simulink model "Lightning_McSeas_VCU_NEW_Speed_Mode"  (R2021b)
settings: Solver=FixedStepDiscrete  StartTime=0.0  StopTime=10.0  FixedStep=0.01  RelTol=1e-3  EnableMultiTasking=on
PreLoadFcn:
  | try, model_open; catch, disp('Error occurred while executing model pre-load callback: model_open.m'); disp('Please assure that the MATLAB working directory is set to the model directory before opening.'); end
InitFcn:
  | try, model_open; catch, end
undefined symbols (not defined in the file): dataName, enumName, enumValue, GCM, raptor_get_safe_string
libraries: Raptor_lib x71, simulink x8
(part 2 of 3)

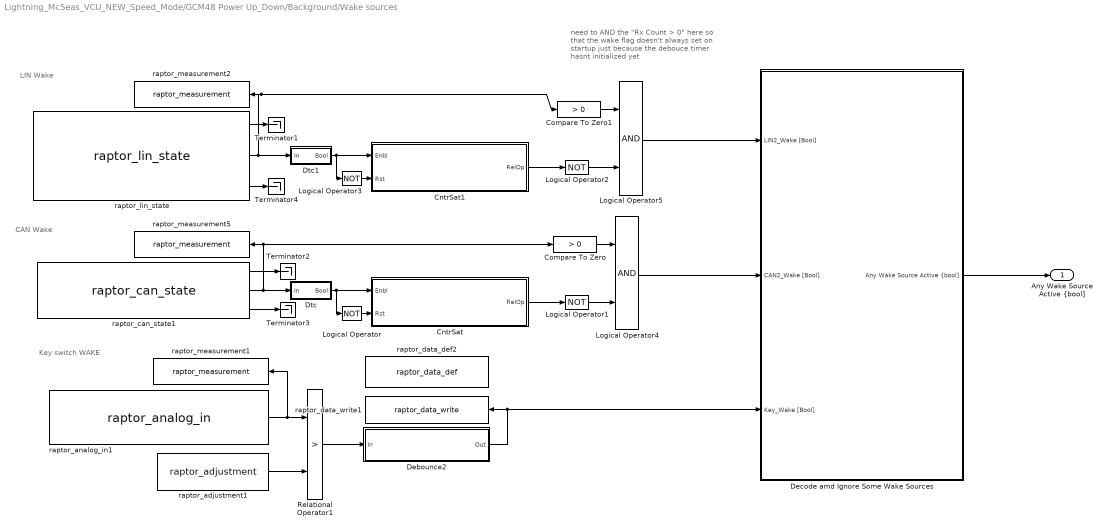
== system Lightning_McSeas_VCU_NEW_Speed_Mode/GCM48 Power Up_Down/Background/Wake sources ==
  note: CAN Wake
  note: Key switch WAKE
  note: LIN Wake
  note: need to AND the "Rx Count > 0" here so that the wake flag doesn't always set on startup just because the debouce timer hasnt initialized yet
  CntrSat : Subsystem  mask(CntrSat){init=0, inc=1, typ=uint32, relop=>=, th_nam='Wake_CAN2_SleepDelayTime', th_help='make sure this is long enough that we dont trigger a ton of EEPROM writes between messages', th_units='sec', th_gain=samptime, th_group=group}
      mask prompts: init "Initial Value (after a reset)"; inc "Increment"; typ "Data Type"; relop "Relational Operator"; th_nam "Thresh. Name"; th_help "Thresh. Help Text"; th_units "Thresh. Units"; th_gain "Thresh. Gain"; th_group "Thresh. Group"
      mask init: same as Lightning_McSeas_VCU_NEW_Speed_Mode/GCM48 Power Up_Down/Background/CntrSat2
      mask TypeOptions typ: double | single | int8 | uint8 | int16 | uint16 | int32 | uint32 | boolean
      mask TypeOptions relop: == | >= | >
      mask Display: disp(['Counter\n' typ '\n' relop ' ' th_nam]);
  CntrSat1 : Subsystem  mask(CntrSat){init=0, inc=1, typ=uint32, relop=>=, th_nam='Wake_LIN2_SleepDelayTime', th_help='make sure this is long enough that we dont trigger a ton of EEPROM writes between messages', th_units='sec', th_gain=samptime, th_group=group}
      mask prompts: init "Initial Value (after a reset)"; inc "Increment"; typ "Data Type"; relop "Relational Operator"; th_nam "Thresh. Name"; th_help "Thresh. Help Text"; th_units "Thresh. Units"; th_gain "Thresh. Gain"; th_group "Thresh. Group"
      mask init: same as Lightning_McSeas_VCU_NEW_Speed_Mode/GCM48 Power Up_Down/Background/CntrSat2
      mask TypeOptions typ: double | single | int8 | uint8 | int16 | uint16 | int32 | uint32 | boolean
      mask TypeOptions relop: == | >= | >
      mask Display: disp(['Counter\n' typ '\n' relop ' ' th_nam]);
  Compare To Zero : simulink/Logic and Bit Operations/Compare To Zero  relop=>  OutDataTypeStr=boolean
  Compare To Zero1 : simulink/Logic and Bit Operations/Compare To Zero  relop=>  OutDataTypeStr=boolean
  Debounce2 : Subsystem
  Decode amd Ignore Some Wake Sources : Subsystem
  Dtc : Subsystem  mask(Dtc){init=0, relop===}
      mask prompts: init "Initial Condition (of input):"; relop "Relational Operator"
      mask init:
      | cb = gcb;
      | 
      | % --- Parameter Setting
      | set_param([cb '/Relational Operator'], 'Operator', relop);
      mask TypeOptions relop: == | ~= | < | <= | >= | >
      mask Display: disp(['U ' relop ' U/z']);
  Dtc1 : Subsystem  mask(Dtc){init=0, relop===}
      mask prompts: init "Initial Condition (of input):"; relop "Relational Operator"
      mask init:
      | cb = gcb;
      | 
      | % --- Parameter Setting
      | set_param([cb '/Relational Operator'], 'Operator', relop);
      mask TypeOptions relop: == | ~= | < | <= | >= | >
      mask Display: disp(['U ' relop ' U/z']);
  Logical Operator{,1..3} (4 alike) : Logic  Operator=NOT  AllPortsSameDT=off  OutDataTypeStr=boolean
  Logical Operator4 : Logic  AllPortsSameDT=off  OutDataTypeStr=boolean
  Logical Operator5 : Logic  AllPortsSameDT=off  OutDataTypeStr=boolean
  Relational Operator1 : RelationalOperator  Operator=>  OutDataTypeStr=boolean  RndMeth=Simplest
  Terminator{1..4} (4 alike) : Terminator
  raptor_adjustment1 : Raptor_lib/Data Storage/raptor_adjustment  paramName='WAKE_INPUT1_Threshold'  nameSource=Parameter  initValue=1200  dataType=uint16  storage=NonVolatile (EEPROM)  calDispType=Number  calEnum={'False', 'True'}  calGain=1  calOffset=0.0  calMax=inf  calMin=-inf  calFormat='-1'  calUnit='V'  calHelp='The value of WAKE_INPUT1 analog to set key switch to true.'  calAccess=4  calFunction=group  calDispHeaders=off  calColHeaders={'Col1' 'Col2' 'Col3'}  calRowHeaders={'Row1' 'Row2' 'Row3'}
      settings: SourceProductName=Raptor
  raptor_analog_in1 : Raptor_lib/Input & Output/raptor_analog_in  resourceValues=DG1|DG2|DG3|DG4|AN1|AN2|AN3|AN4|AN5|AN6|AN7|AN8|AN9|AN10|AN11|AN12|WAKE_INPUT1|(None)  resource=WAKE_INPUT1  pullUDValues=[]  pullUD=[]  rangeValues=[]  range=[]  filterrateValues=[]  filterrate='RAPTOR MASK DEFAULT'  resolutionValues=[]  resolution=[]
      settings: SourceProductName=Raptor
  raptor_can_state1 : Raptor_lib/CAN/raptor_can_state  resourceValues=CAN1|CAN2|CAN3|CAN4|CAN5|CAN6|(None)  resource=CAN2  errOut='RAPTOR MASK DEFAULT'
      settings: SourceProductName=Raptor
  raptor_data_def2 : Raptor_lib/Data Storage/raptor_data_def  dataName='KeySw_Bgnd'  initValue=0  dataType=boolean  storage=Volatile (RAM)  calVisible=on  calType=Measurement  calDispType=Number  calEnum={'False', 'True'}  calGain=1.0  calOffset=0  calMin=-Inf  calMax=Inf  calFormat='-1'  calUnit='Bool'  calHelp='Key switch reading from background task'  calAccess=4  calFunction=group  calDispHeaders=off  calColHeaders={'Col1' 'Col2' 'Col3'}  calRowHeaders={'Row1' 'Row2' 'Row3'}
      settings: SourceProductName=Raptor
  raptor_data_write1 : Raptor_lib/Data Storage/raptor_data_write  dataName='KeySw_Bgnd'  dataShape=Scalar  idxSource=Input Port  idxRow=1  idxCol=1
      settings: SourceProductName=Raptor
  raptor_lin_state : Raptor_lib/LIN/raptor_lin_state  linBus='LIN2'
      settings: SourceProductName=Raptor
  raptor_measurement1 : Raptor_lib/Data Storage/raptor_measurement  paramName='Wake_INPUT1_Vlts'  nameSource=Parameter  calDispType=Number  calEnum={'False', 'True'}  calGain=38/4096  calOffset=0.0  calMax=inf  calMin=-inf  calFormat='-1'  calUnit=''  calHelp=''  calAccess=4  calFunction=group  calVisible=on
      settings: SourceProductName=Raptor
  raptor_measurement2 : Raptor_lib/Data Storage/raptor_measurement  paramName='Wake_LIN2_RxCount'  nameSource=Parameter  calDispType=Number  calEnum={'False', 'True'}  calGain=1.0  calOffset=0.0  calMax=inf  calMin=-inf  calFormat='-1'  calUnit=''  calHelp=''  calAccess=4  calFunction=group  calVisible=on
      settings: SourceProductName=Raptor
  raptor_measurement5 : Raptor_lib/Data Storage/raptor_measurement  paramName='Wake_CAN2_RxCount'  nameSource=Parameter  calDispType=Number  calEnum={'False', 'True'}  calGain=1.0  calOffset=0.0  calMax=inf  calMin=-inf  calFormat='-1'  calUnit=''  calHelp=''  calAccess=4  calFunction=group  calVisible=on
      settings: SourceProductName=Raptor
  "Any Wake Source Active {bool]" : Outport  VectorParamsAs1DForOutWhenUnconnected=off
  wires:
  Logical Operator5/1 -> Decode amd Ignore Some Wake Sources/1(LIN2_Wake [Bool])
  Logical Operator2/1 -> Logical Operator5/2
  Compare To Zero1/1 -> Logical Operator5/1
  Logical Operator4/1 -> Decode amd Ignore Some Wake Sources/2(CAN2_Wake [Bool])
  Compare To Zero/1 -> Logical Operator4/1
  Logical Operator1/1 -> Logical Operator4/2
  Decode amd Ignore Some Wake Sources/1("Any Wake Source Active {bool]") -> "Any Wake Source Active {bool]"/1
  raptor_can_state1/3 -> Terminator3/1
  raptor_adjustment1/1 -> Relational Operator1/2
  raptor_can_state1/1 -> Terminator2/1
  raptor_lin_state/3 -> Terminator4/1
  raptor_lin_state/1 -> Terminator1/1
  CntrSat1/1(RelOp) -> Logical Operator2/1
  Logical Operator/1 -> CntrSat/2(Rst)
  raptor_lin_state/2 -> Dtc1/1(In), raptor_measurement2/1, Compare To Zero1/1
  Logical Operator3/1 -> CntrSat1/2(Rst)
  Dtc1/1(Bool) -> Logical Operator3/1, CntrSat1/1(Enbl)
  Relational Operator1/1 -> Debounce2/1(In)
  Dtc/1(Bool) -> CntrSat/1(Enbl), Logical Operator/1
  CntrSat/1(RelOp) -> Logical Operator1/1
  raptor_analog_in1/1 -> Relational Operator1/1, raptor_measurement1/1
  Debounce2/1(Out) -> raptor_data_write1/1, Decode amd Ignore Some Wake Sources/3(Key_Wake [Bool])
  raptor_can_state1/2 -> raptor_measurement5/1, Compare To Zero/1, Dtc/1(In)

== system Lightning_McSeas_VCU_NEW_Speed_Mode/Foreground/CAN/RC Rx/Actuators ==
  note: This subsystem isnt correct****
  note: -might be able to just combine back actuators to same thing - or they might be inversers of each other
  Rise of Back : Inport
  Rise of Front : Inport  Port=2
  Gain1 : Gain  Gain=51
  Gain2 : Gain  Gain=51
  If statement for on off switch1 : Subsystem  Commented=on
  Subsystem : Subsystem  Commented=on
  raptor_can_txmsg3 : Raptor_lib/CAN/raptor_can_txmsg  canDefinition=struct('dbcFile', 'actuator_atmpt1.dbc','message', 'actuator3','comment', '','signals', {{'position_send3'}},'enabled', [ 1;],'scaled', [ 1;],'canBus', '''CAN1''','messageID', [ 32;],'idMask', [ 536870911;],'payloadMask', [],'payloadValue', [],'period', [ 0;],'mailbox', '','queueSize', [ 1;],'label', [ 0;],'ver', [ 2;],'showID', [ 0;],'showRaw', [ 0;],'showRawMsg', [ 0;],'fill', [ 0;],'editID', [ 0;],'signalOrder', [ 1;],'signalAscDes', [ 1;])  canBus='CAN1'  queueSize=1  payloadMask=[]  payloadValue=[]  period=0  showID=0  label=0  idMask=hex2dec('1FFFFFFF')  fill=0  id=32  showRaw=0  signalOrder=1  signalInfo={{struct('Name', 'position_send3','Startbit', [ 0;],'SignalSize', [ 16;],'ByteOrder', 'LittleEndian','ValueType', 'UNSIGNED','Class', 'uint16','Signed', [ 0;],'Factor', [ 1;],'Offset', [ 0;],'Min', [ 0;],'Max', [ 0;],'Units', '','Comment', '','StartBit', [ 0;])}}
      settings: SourceProductName=Raptor
  raptor_can_txmsg4 : Raptor_lib/CAN/raptor_can_txmsg  canDefinition=struct('dbcFile', 'actuator_atmpt1.dbc','message', 'actuator2','comment', '','signals', {{'position_send2'}},'enabled', [ 1;],'scaled', [ 1;],'canBus', '''CAN1''','messageID', [ 31;],'idMask', [ 536870911;],'payloadMask', [],'payloadValue', [],'period', [ 0;],'mailbox', '','queueSize', [ 1;],'label', [ 0;],'ver', [ 2;],'showID', [ 0;],'showRaw', [ 0;],'showRawMsg', [ 0;],'fill', [ 0;],'editID', [ 0;],'signalOrder', [ 1;],'signalAscDes', [ 1;])  canBus='CAN1'  queueSize=1  payloadMask=[]  payloadValue=[]  period=0  showID=0  label=0  idMask=hex2dec('1FFFFFFF')  fill=0  id=31  showRaw=0  signalOrder=1  signalInfo={{struct('Name', 'position_send2','Startbit', [ 0;],'SignalSize', [ 16;],'ByteOrder', 'LittleEndian','ValueType', 'UNSIGNED','Class', 'uint16','Signed', [ 0;],'Factor', [ 1;],'Offset', [ 0;],'Min', [ 0;],'Max', [ 0;],'Units', '','Comment', '','StartBit', [ 0;])}}
      settings: SourceProductName=Raptor
  wires:
  Rise of Back/1 -> Gain2/1
  Gain2/1 -> raptor_can_txmsg4/1
  Gain1/1 -> raptor_can_txmsg3/1
  Rise of Front/1 -> Gain1/1

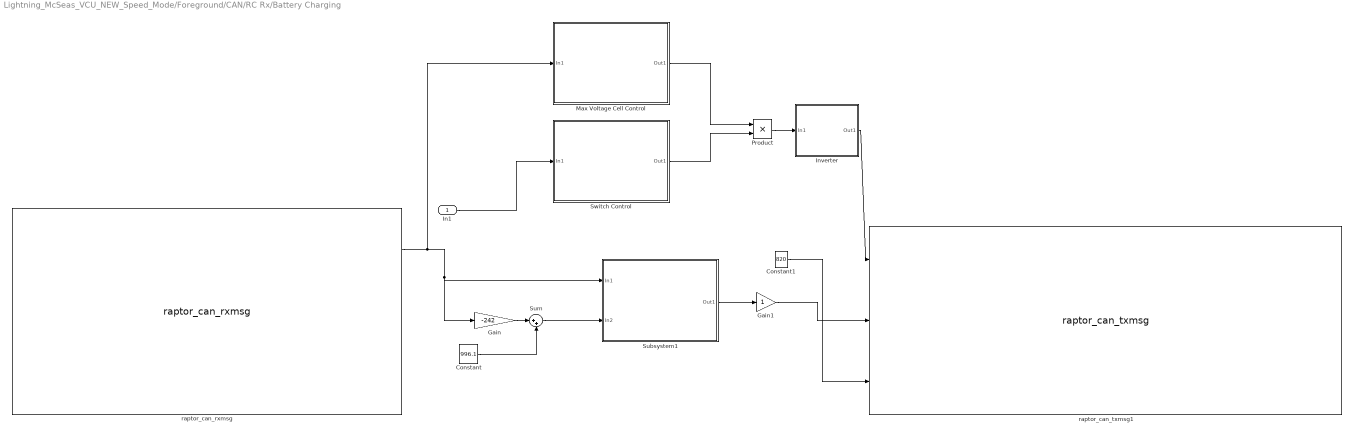
== system Lightning_McSeas_VCU_NEW_Speed_Mode/Foreground/CAN/RC Rx/Battery Charging ==
  In1 : Inport
  Constant : Constant  Value=996.1
  Constant1 : Constant  Value=820
  Gain : Gain  Gain=-242
  Gain1 : Gain
  Inverter : Subsystem
  Max Voltage Cell Control : Subsystem
  Product : Product
  Subsystem1 : Subsystem
  Sum : Sum  Inputs=|++
  Switch Control : Subsystem
  raptor_can_rxmsg : Raptor_lib/CAN/raptor_can_rxmsg  canDefinition=struct('dbcFile', 'BCM_VehBus_StdInterface.dbc','message', 'BCM_Meas_A','comment', '','signals', {{'bcm_cell_vmax_a','bcm_cell_vmin_a','bcm_i_lem_a','bcm_vbat_a','bcm_vbus_a','bcm_vfuse_a'}},'enabled', [ 1 1 1 1 1 1;],'scaled', [ 1 1 1 1 1 1;],'canBus', '''CAN1''','messageID', [ 1072;],'idMask', [ 536870911;],'payloadMask', [],'payloadValue', [],'period', [ 0;],'mailbox', '''''','queueSize', [ 1;],'label', [ 0;],'ver', [ 2;],'showID', [ 0;],'showRaw', [ 0;],'showRawMsg', [ 0;],'showAge', [ 1;],'fill', [ 0;],'editID', [ 0;],'signalOrder', [ 1;],'signalAscDes', [ 1;])  canBus='CAN1'  mailbox=''  payloadMask=[]  payloadValue=[]  idMask=hex2dec('1FFFFFFF')  queueSize=1  showID=0  label=0  fill=0  id=1072  showRaw=0  showAge=1  signalOrder=1  signalInfo={{struct('Name', 'bcm_cell_vmin_a','Startbit', [ 0;],'SignalSize', [ 12;],'ByteOrder', 'BigEndian','ValueType', 'UNSIGNED','Class', 'uint16','Signed', [ 0;],'Factor', [ 0.002;],'Offset', [ 0;],'Min', [ 0;],'Max', [ 5;],'Units', 'volts','Comment', 'Min cell voltage.','StartBit', [ 56;]),struct('Name', 'bcm_cell_vmax_a','Startbit', [ 0;],'SignalSize', [ 12;],'ByteOrder', 'BigEndian','ValueType', 'UNSIGNED','Class', 'uint16','Signed', [ 0;],'Factor', [ 0.002;],'Offset', [ 0;],'Min', [ 0;],'Max', [ 5;],'Units', 'volts','Comment', 'Max cell voltage.','StartBit', [ 52;]),struct('Name', 'bcm_vfuse_a','Startbit', [ 0;],'SignalSize', [ 8;],'ByteOrder', 'BigEndian','ValueType', 'UNSIGNED','Class', 'uint8','Signed', [ 0;],'Factor', [ 0.5;],'Offset', [ 0;],'Min', [ 0;],'Max', [ 125;],'Units', 'volts','Comment', 'HV bus positive voltage measurement.','StartBit', [ 24;]),struct('Name', 'bcm_vbus_a','Startbit', [ 0;],'SignalSize', [ 8;],'ByteOrder', 'BigEndian','ValueType', 'UNSIGNED','Class', 'uint8','Signed', [ 0;],'Factor', [ 0.5;],'Offset', [ 0;],'Min', [ 0;],'Max', [ 125;],'Units', 'volts','Comment', 'HV bus positive voltage measurement.','StartBit', [ 32;]),struct('Name', 'bcm_vbat_a','Startbit', [ 0;],'SignalSize', [ 8;],'ByteOrder', 'BigEndian','ValueType', 'UNSIGNED','Class', 'uint8','Signed', [ 0;],'Factor', [ 0.5;],'Offset', [ 0;],'Min', [ 0;],'Max', [ 125;],'Units', 'volts','Comment', 'HV bus positive voltage measurement.','StartBit', [ 16;]),struct('Name', 'bcm_i_lem_a','Startbit', [ 0;],'SignalSize', [ 16;],'ByteOrder', 'BigEndian','ValueType', 'UNSIGNED','Class', 'uint16','Signed', [ 0;],'Factor', [ 0.025;],'Offset', [ -1000;],'Min', [ -1000;],'Max', [ 500;],'Units', 'amps','Comment', '[Development Sensor] HV Battery Current where negative is battery discharge and positive is battery charge.','StartBit', [ 8;])}}  showRawMsg=0
      settings: SourceProductName=Raptor
  raptor_can_txmsg1 : Raptor_lib/CAN/raptor_can_txmsg  canDefinition=struct('dbcFile', 'Elcon_Charger.dbc','message', 'Charger_Request','comment', '','signals', {{'charger_control','charger_max_current','charger_max_voltage'}},'enabled', [ 1 1 1;],'scaled', [ 1 1 1;],'canBus', '''CAN1''','messageID', [ 403105268;],'idMask', [ 536870911;],'payloadMask', [],'payloadValue', [],'period', [ 0;],'mailbox', '','queueSize', [ 1;],'label', [ 0;],'ver', [ 2;],'showID', [ 0;],'showRaw', [ 0;],'showRawMsg', [ 0;],'fill', [ 0;],'editID', [ 0;],'signalOrder', [ 1;],'signalAscDes', [ 1;])  canBus='CAN1'  queueSize=1  payloadMask=[]  payloadValue=[]  period=0  showID=0  label=0  idMask=hex2dec('1FFFFFFF')  fill=0  id=403105268  showRaw=0  signalOrder=1  signalInfo={{struct('Name', 'charger_max_voltage','Startbit', [ 0;],'SignalSize', [ 16;],'ByteOrder', 'BigEndian','ValueType', 'UNSIGNED','Class', 'uint16','Signed', [ 0;],'Factor', [ 0.1;],'Offset', [ 0;],'Min', [ 0;],'Max', [ 0;],'Units', 'V','Comment', 'Max Allowable Charging Terminal Voltage','StartBit', [ 8;]),struct('Name', 'charger_max_current','Startbit', [ 0;],'SignalSize', [ 16;],'ByteOrder', 'BigEndian','ValueType', 'UNSIGNED','Class', 'uint16','Signed', [ 0;],'Factor', [ 0.1;],'Offset', [ 0;],'Min', [ 0;],'Max', [ 0;],'Units', 'A','Comment', 'Max Allowable Charging Current','StartBit', [ 24;]),struct('Name', 'charger_control','Startbit', [ 0;],'SignalSize', [ 8;],'ByteOrder', 'LittleEndian','ValueType', 'UNSIGNED','Class', 'uint8','Signed', [ 0;],'Factor', [ 1;],'Offset', [ 0;],'Min', [ 0;],'Max', [ 0;],'Units', '','Comment', 'Toggle charging','StartBit', [ 32;])}}
      settings: SourceProductName=Raptor
  wires:
  In1/1 -> Switch Control/1(In1)
  Gain/1 -> Sum/1
  Subsystem1/1(Out1) -> Gain1/1
  Constant1/1 -> raptor_can_txmsg1/3
  Constant/1 -> Sum/2
  Sum/1 -> Subsystem1/2(In2)
  Switch Control/1(Out1) -> Product/2
  Max Voltage Cell Control/1(Out1) -> Product/1
  Gain1/1 -> raptor_can_txmsg1/2
  raptor_can_rxmsg/2 -> Max Voltage Cell Control/1(In1), Gain/1, Subsystem1/1(In1)
  Product/1 -> Inverter/1(In1)
  Inverter/1(Out1) -> raptor_can_txmsg1/1

== system Lightning_McSeas_VCU_NEW_Speed_Mode/Foreground/CAN/RC Rx/Battery Switch ==
  value in : Inport
  Constant : Constant  Commented=on  Value=10000  OutDataTypeStr=uint16
  Constant1 : Constant  Commented=on  Value=100  OutDataTypeStr=uint32
  If statement for on off switch : Subsystem
  If statement for on off switch1 : Subsystem  Commented=on
  If statement for on off switch2 : Subsystem
  raptor_can_txmsg : Raptor_lib/CAN/raptor_can_txmsg  canDefinition=struct('dbcFile', 'BCM_VehBus_StdInterface.dbc','message', 'BCM_Request','comment', '','signals', {{'hsc_bcm_enable','hsc_bcm_epo','hsc_bcm_leakage_ena','hsc_bcm_mainc_close'}},'enabled', [ 1 1 1 1;],'scaled', [ 1 1 1 1;],'canBus', '''CAN1''','messageID', [ 1024;],'idMask', [ 536870911;],'payloadMask', [],'payloadValue', [],'period', [ 0;],'mailbox', '','queueSize', [ 1;],'label', [ 0;],'ver', [ 2;],'showID', [ 0;],'showRaw', [ 0;],'showRawMsg', [ 0;],'fill', [ 0;],'editID', [ 0;],'signalOrder', [ 1;],'signalAscDes', [ 1;])  canBus='CAN1'  queueSize=1  payloadMask=[]  payloadValue=[]  period=0  showID=0  label=0  idMask=hex2dec('1FFFFFFF')  fill=0  id=1024  showRaw=0  signalOrder=1  signalInfo={{struct('Name', 'hsc_bcm_mainc_close','Startbit', [ 0;],'SignalSize', [ 1;],'ByteOrder', 'BigEndian','ValueType', 'UNSIGNED','Class', 'uint8','Signed', [ 0;],'Factor', [ 1;],'Offset', [ 0;],'Min', [ 0;],'Max', [ 1;],'Units', 'flag','Comment', 'Vehicle main contactor command.','StartBit', [ 2;]),struct('Name', 'hsc_bcm_leakage_ena','Startbit', [ 0;],'SignalSize', [ 1;],'ByteOrder', 'BigEndian','ValueType', 'UNSIGNED','Class', 'uint8','Signed', [ 0;],'Factor', [ 1;],'Offset', [ 0;],'Min', [ 0;],'Max', [ 1;],'Units', 'flag','Comment', 'Vehicle leakage detection enabled (bcm_gfd calculation).','StartBit', [ 3;]),struct('Name', 'hsc_bcm_epo','Startbit', [ 0;],'SignalSize', [ 1;],'ByteOrder', 'BigEndian','ValueType', 'UNSIGNED','Class', 'uint8','Signed', [ 0;],'Factor', [ 1;],'Offset', [ 0;],'Min', [ 0;],'Max', [ 1;],'Units', 'flag','Comment', 'Vehicle Emergency Power Off command, fast shutdown.','StartBit', [ 1;]),struct('Name', 'hsc_bcm_enable','Startbit', [ 0;],'SignalSize', [ 1;],'ByteOrder', 'BigEndian','ValueType', 'UNSIGNED','Class', 'uint8','Signed', [ 0;],'Factor', [ 1;],'Offset', [ 0;],'Min', [ 0;],'Max', [ 1;],'Units', 'flag','Comment', 'Flag from vehicle controller allowing BCM to accept commands.','StartBit', [ 0;])}}
      settings: SourceProductName=Raptor
  raptor_pwm_out : Raptor_lib/Input & Output/raptor_pwm_out  Commented=on  showEnable=1  resourceValues=LSO1|LSO2|LSO3|LSO4|LSO5|LSO6|LSO7|LSO8|(None)  resource=LSO2  driverTypeValues=Low Side  driverType=Low Side
      settings: SourceProductName=Raptor
  wires:
  value in/1 -> If statement for on off switch2/1(value in), If statement for on off switch/1(value in)
  If statement for on off switch2/1(Value out) -> raptor_can_txmsg/1
  If statement for on off switch1/1(Value out) -> raptor_pwm_out/1
  Constant1/1 -> raptor_pwm_out/3
  Constant/1 -> raptor_pwm_out/2
  If statement for on off switch/1(Value out) -> raptor_can_txmsg/4

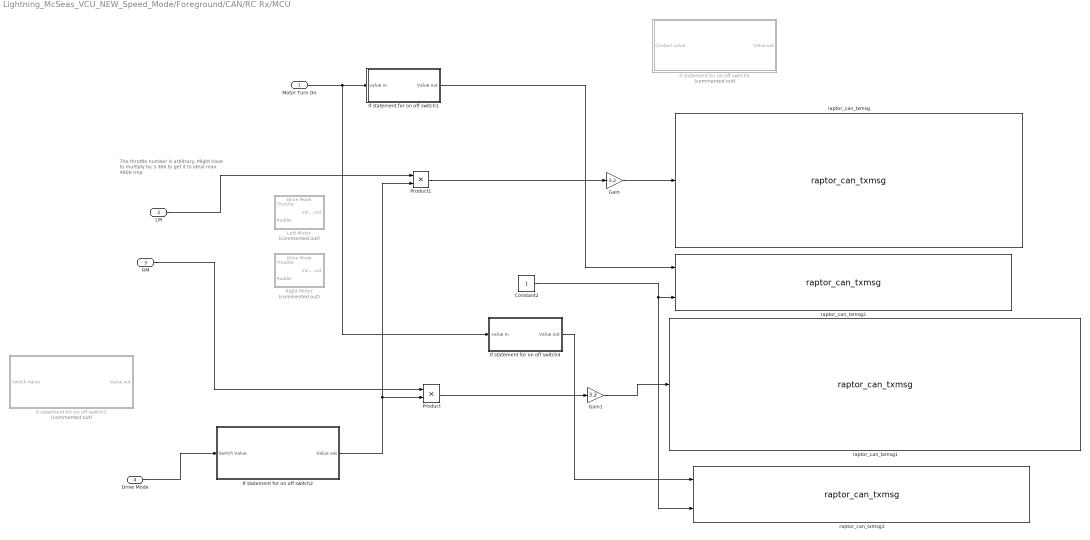
== system Lightning_McSeas_VCU_NEW_Speed_Mode/Foreground/CAN/RC Rx/MCU ==
  note: The throttle number is arbitrary. Might have to multiply by 3.366 to get it to ideal max 4800 rmp
  Motor Turn On : Inport
  LM : Inport  Port=2
  RM : Inport  Port=3
  Drive Mode : Inport  Port=4
  Constant2 : Constant
  Gain : Gain  Gain=-3.2
  Gain1 : Gain  Gain=3.2
  If statement for on off switch1 : Subsystem
  If statement for on off switch2 : Subsystem
  If statement for on off switch3 : Subsystem  Commented=on
  If statement for on off switch4 : Subsystem
  If statement for on off switch5 : Subsystem  Commented=on
  Left Motor : Subsystem  Commented=on
      settings: PortSchema="{\"entries\":[{\"content\":{\"sides\":[{\"content\":{\"connectorIds\":[\"In1\",\"In2\"]},\"type\":\"ConnectorPlacement.EquallySpacedRectSide\",\"uuid\":\"2083280e-5025-4497-a6f4-d95150e30dec\"},{\"content\":{\"connectorIds\":[\"Out1\"],\"side\":\"RIGHT\"},\"type\":\"ConnectorPlacement.EquallySpacedRectSide\",\"uuid\":\"61c851a0-d108-4419-a7df-f59beb96b75c\"},{\"content\":{\"connectorIds\":[\"In3\"],\"side\":\"TOP\"},\"type\":\"ConnectorPlacement.EquallySpacedRectSide\",\"uuid\":\"d9cef341-ca3e-4785-954e-89a8b6a8f97d\"}]},\"type\":\"ConnectorPlacement.EquallySpacedConnector\",\"uuid\":\"5877ad35-291b-4063-ae6a-1f18cb91c1ea\"}],\"packageUris\":[\"http://schema.mathworks.com/mf0/Connector/R2020b\"],\"version\":\"1.0\"}"
  Product : Product
  Product1 : Product
  Right Motor : Subsystem  Commented=on
      settings: PortSchema="{\"entries\":[{\"content\":{\"sides\":[{\"content\":{\"connectorIds\":[\"In1\",\"In2\"]},\"type\":\"ConnectorPlacement.EquallySpacedRectSide\",\"uuid\":\"2083280e-5025-4497-a6f4-d95150e30dec\"},{\"content\":{\"connectorIds\":[\"Out1\"],\"side\":\"RIGHT\"},\"type\":\"ConnectorPlacement.EquallySpacedRectSide\",\"uuid\":\"61c851a0-d108-4419-a7df-f59beb96b75c\"},{\"content\":{\"connectorIds\":[\"In3\"],\"side\":\"TOP\"},\"type\":\"ConnectorPlacement.EquallySpacedRectSide\",\"uuid\":\"d9cef341-ca3e-4785-954e-89a8b6a8f97d\"}]},\"type\":\"ConnectorPlacement.EquallySpacedConnector\",\"uuid\":\"5877ad35-291b-4063-ae6a-1f18cb91c1ea\"}],\"packageUris\":[\"http://schema.mathworks.com/mf0/Connector/R2020b\"],\"version\":\"1.0\"}"
  raptor_can_txmsg : Raptor_lib/CAN/raptor_can_txmsg  canDefinition=struct('dbcFile', 'A1_MICH_EV_BOAT.dbc','message', 'command1','comment', '','signals', {{'throttleCurrent1'}},'enabled', [ 1;],'scaled', [ 1;],'canBus', '''CAN1''','messageID', [ 550;],'idMask', [ 536870911;],'payloadMask', [],'payloadValue', [],'period', [ 0;],'mailbox', '','queueSize', [ 1;],'label', [ 0;],'ver', [ 2;],'showID', [ 0;],'showRaw', [ 0;],'showRawMsg', [ 0;],'fill', [ 0;],'editID', [ 0;],'signalOrder', [ 1;],'signalAscDes', [ 1;])  canBus='CAN1'  queueSize=1  payloadMask=[]  payloadValue=[]  period=0  showID=0  label=0  idMask=hex2dec('1FFFFFFF')  fill=0  id=550  showRaw=0  signalOrder=1  signalInfo={{struct('Name', 'throttleCurrent1','Startbit', [ 0;],'SignalSize', [ 16;],'ByteOrder', 'LittleEndian','ValueType', 'SIGNED','Class', 'int16','Signed', [ 1;],'Factor', [ 1;],'Offset', [ 0;],'Min', [ 0;],'Max', [ 0;],'Units', '','Comment', '','StartBit', [ 0;])}}
      settings: SourceProductName=Raptor
  raptor_can_txmsg1 : Raptor_lib/CAN/raptor_can_txmsg  canDefinition=struct('dbcFile', 'A1_MICH_EV_BOAT.dbc','message', 'command1','comment', '','signals', {{'throttleCurrent1'}},'enabled', [ 1;],'scaled', [ 1;],'canBus', '''CAN1''','messageID', [ 550;],'idMask', [ 536870911;],'payloadMask', [],'payloadValue', [],'period', [ 0;],'mailbox', '','queueSize', [ 1;],'label', [ 0;],'ver', [ 2;],'showID', [ 0;],'showRaw', [ 0;],'showRawMsg', [ 0;],'fill', [ 0;],'editID', [ 0;],'signalOrder', [ 1;],'signalAscDes', [ 1;])  canBus='CAN1'  queueSize=1  payloadMask=[]  payloadValue=[]  period=0  showID=0  label=0  idMask=hex2dec('1FFFFFFF')  fill=0  id=550  showRaw=0  signalOrder=1  signalInfo={{struct('Name', 'throttleCurrent1','Startbit', [ 0;],'SignalSize', [ 16;],'ByteOrder', 'LittleEndian','ValueType', 'SIGNED','Class', 'int16','Signed', [ 1;],'Factor', [ 1;],'Offset', [ 0;],'Min', [ 0;],'Max', [ 0;],'Units', '','Comment', '','StartBit', [ 0;])}}
      settings: SourceProductName=Raptor
  raptor_can_txmsg2 : Raptor_lib/CAN/raptor_can_txmsg  canDefinition=struct('dbcFile', 'A1_MICH_EV_BOAT.dbc','message', 'NMT','comment', '','signals', {{'id','o1'}},'enabled', [ 1 1;],'scaled', [ 1 1;],'canBus', '''CAN1''','messageID', [ 0;],'idMask', [ 536870911;],'payloadMask', [],'payloadValue', [],'period', [ 0;],'mailbox', '','queueSize', [ 1;],'label', [ 0;],'ver', [ 2;],'showID', [ 0;],'showRaw', [ 0;],'showRawMsg', [ 0;],'fill', [ 0;],'editID', [ 0;],'signalOrder', [ 1;],'signalAscDes', [ 1;])  canBus='CAN1'  queueSize=1  payloadMask=[]  payloadValue=[]  period=0  showID=0  label=0  idMask=hex2dec('1FFFFFFF')  fill=0  id=0  showRaw=0  signalOrder=1  signalInfo={{struct('Name', 'id','Startbit', [ 0;],'SignalSize', [ 8;],'ByteOrder', 'LittleEndian','ValueType', 'UNSIGNED','Class', 'uint8','Signed', [ 0;],'Factor', [ 1;],'Offset', [ 0;],'Min', [ 0;],'Max', [ 0;],'Units', '','Comment', 'controller id hex (0x26 or 0x27 in our case)','StartBit', [ 8;]),struct('Name', 'o1','Startbit', [ 0;],'SignalSize', [ 8;],'ByteOrder', 'LittleEndian','ValueType', 'UNSIGNED','Class', 'uint8','Signed', [ 0;],'Factor', [ 1;],'Offset', [ 0;],'Min', [ 0;],'Max', [ 0;],'Units', '','Comment', 'value 01 hex','StartBit', [ 0;])}}
      settings: SourceProductName=Raptor
  raptor_can_txmsg3 : Raptor_lib/CAN/raptor_can_txmsg  canDefinition=struct('dbcFile', 'A1_MICH_EV_BOAT.dbc','message', 'NMT','comment', '','signals', {{'id','o1'}},'enabled', [ 1 1;],'scaled', [ 1 1;],'canBus', '''CAN1''','messageID', [ 0;],'idMask', [ 536870911;],'payloadMask', [],'payloadValue', [],'period', [ 0;],'mailbox', '','queueSize', [ 1;],'label', [ 0;],'ver', [ 2;],'showID', [ 0;],'showRaw', [ 0;],'showRawMsg', [ 0;],'fill', [ 0;],'editID', [ 0;],'signalOrder', [ 1;],'signalAscDes', [ 1;])  canBus='CAN1'  queueSize=1  payloadMask=[]  payloadValue=[]  period=0  showID=0  label=0  idMask=hex2dec('1FFFFFFF')  fill=0  id=0  showRaw=0  signalOrder=1  signalInfo={{struct('Name', 'id','Startbit', [ 0;],'SignalSize', [ 8;],'ByteOrder', 'LittleEndian','ValueType', 'UNSIGNED','Class', 'uint8','Signed', [ 0;],'Factor', [ 1;],'Offset', [ 0;],'Min', [ 0;],'Max', [ 0;],'Units', '','Comment', 'controller id hex (0x26 or 0x27 in our case)','StartBit', [ 8;]),struct('Name', 'o1','Startbit', [ 0;],'SignalSize', [ 8;],'ByteOrder', 'LittleEndian','ValueType', 'UNSIGNED','Class', 'uint8','Signed', [ 0;],'Factor', [ 1;],'Offset', [ 0;],'Min', [ 0;],'Max', [ 0;],'Units', '','Comment', 'value 01 hex','StartBit', [ 0;])}}
      settings: SourceProductName=Raptor
  wires:
  Motor Turn On/1 -> If statement for on off switch4/1(value in), If statement for on off switch1/1(value in)
  RM/1 -> Product/1
  LM/1 -> Product1/1
  Product/1 -> Gain1/1
  Product1/1 -> Gain/1
  If statement for on off switch2/1(Value out) -> Product1/2, Product/2
  Drive Mode/1 -> If statement for on off switch2/1(Switch Value)
  Gain/1 -> raptor_can_txmsg/1
  Gain1/1 -> raptor_can_txmsg1/1
  If statement for on off switch1/1(Value out) -> raptor_can_txmsg2/1
  Constant2/1 -> raptor_can_txmsg3/2, raptor_can_txmsg2/2
  If statement for on off switch4/1(Value out) -> raptor_can_txmsg3/1

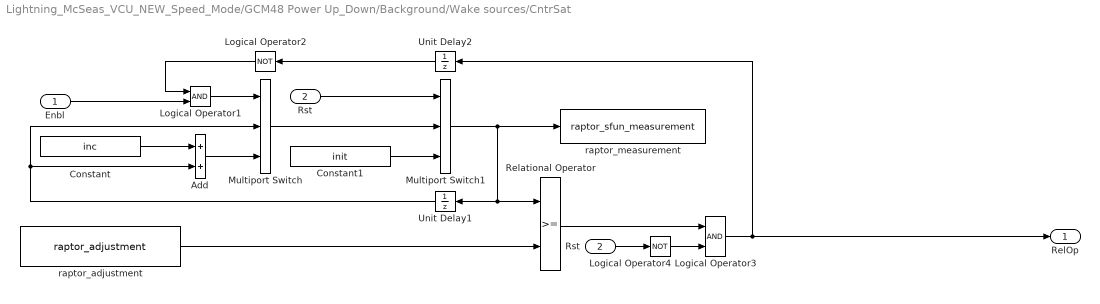
== system Lightning_McSeas_VCU_NEW_Speed_Mode/GCM48 Power Up_Down/Background/Wake sources/CntrSat ==
  Enbl : Inport
  Rst : Inport  Port=2
  Add : Sum  InputSameDT=on  OutDataTypeStr=Inherit: Same as first input
  Constant : Constant  Value=inc  OutDataTypeStr=uint32
  Constant1 : Constant  Value=init  OutDataTypeStr=uint32
  Logical Operator1 : Logic  OutDataTypeStr=boolean
  Logical Operator2 : Logic  Operator=NOT  Inputs=1  OutDataTypeStr=boolean
  Logical Operator3 : Logic  OutDataTypeStr=boolean
  Logical Operator4 : Logic  Operator=NOT  Inputs=1  OutDataTypeStr=boolean
  Multiport Switch : MultiPortSwitch  DataPortOrder=Zero-based contiguous  Inputs=2  zeroidx=on  InputSameDT=on
  Multiport Switch1 : MultiPortSwitch  DataPortOrder=Zero-based contiguous  Inputs=2  zeroidx=on  InputSameDT=on
  Relational Operator : RelationalOperator  OutDataTypeStr=boolean  RndMeth=Nearest
  "Rst " : InportShadow  Port=2
  Unit Delay1 : UnitDelay  InitialCondition=init  SampleTime=-1  HasFrameUpgradeWarning=on
  Unit Delay2 : UnitDelay  InitialCondition=boolean(0)  SampleTime=-1  HasFrameUpgradeWarning=on
  raptor_adjustment : Raptor_lib/Data Storage/raptor_adjustment  paramName=th_nam  nameSource=Parameter  initValue=5 / th_gain  dataType=uint32  storage=Calibration  calDispType=Number  calEnum={'Disabled', 'Enabled'}  calGain=th_gain  calOffset=0  calMax=inf  calMin=-inf  calFormat='0.3'  calUnit=th_units  calHelp=th_help  calAccess=4  calFunction=th_group  calDispHeaders=off  calColHeaders={'Col1' 'Col2' 'Col3'}  calRowHeaders={'Row1' 'Row2' 'Row3'}
      settings: SourceProductName=Raptor
  raptor_measurement : S-Function  FunctionName=raptor_sfun_measurement  Parameters=char({dataName,''}), uint8(calDispType), char(enumName), int32(enumValue), double(calGain), double(calOffset), double(calMax), double(calMin), char(calUnit), char(calHelp), char(calFormat), char(calFunction), char(calAccess)  SFunctionDeploymentMode=off  EnableBusSupport=off  mask(Measurement){paramName=[th_nam(1:end-3) 'Tmr'], nameSource=Parameter, calDispType=Number, calEnum={'False', 'True'}, calGain=th_gain, calOffset=0.0, calMax=inf, calMin=-inf, calFormat='0.3', calUnit=th_units, calHelp=['time that gets compared to ' th_nam], calAccess=4, calFunction=th_group, calVisible=on}
      mask prompts: paramName "Name"; nameSource "Name Source"; calDispType "Display as"; calEnum "Enumeration Definition"; calGain "Gain"; calOffset "Offset"; calMax "Max"; calMin "Min"; calFormat "Display Decimal Places"; calUnit "Unit Text"; calHelp "Help Text"; calAccess "Access Level"; calFunction "Function"; calVisible "Visible in Cal"
      mask help: This block is used to display a value in the calibration tool.
      mask init:
      | raptor_sfun_measurement_maskInit;
      settings: MoveFcn=raptor_icon_redraw(gcb);
      mask Help: eval('raptor_help(''raptor_measurement'');')
      mask TypeOptions nameSource: Parameter | Input Wire
      mask Callback nameSource: raptor_sfun_measurement_dlgCb(gcb, 'nameSource');
      mask TypeOptions calDispType: Number | Enumeration | String
      mask Callback calDispType: raptor_sfun_measurement_dlgCb(gcb, 'calDispType');
      mask TypeOptions calAccess: 4 | 3 | 2 | 1
      mask Display: raptor_sfun_measurement_icon;
  RelOp : Outport  VectorParamsAs1DForOutWhenUnconnected=off
  wires:
  Unit Delay2/1 -> Logical Operator2/1
  Rst/1 -> Multiport Switch1/1
  Logical Operator3/1 -> Unit Delay2/1, RelOp/1
  raptor_adjustment/1 -> Relational Operator/2
  Enbl/1 -> Logical Operator1/2
  Logical Operator1/1 -> Multiport Switch/1
  Add/1 -> Multiport Switch/3
  Unit Delay1/1 -> Add/2, Multiport Switch/2
  Constant/1 -> Add/1
  Multiport Switch/1 -> Multiport Switch1/2
  Constant1/1 -> Multiport Switch1/3
  Logical Operator2/1 -> Logical Operator1/1
  Multiport Switch1/1 -> raptor_measurement/1, Unit Delay1/1, Relational Operator/1
  Relational Operator/1 -> Logical Operator3/1
  Logical Operator4/1 -> Logical Operator3/2
  "Rst "/1 -> Logical Operator4/1

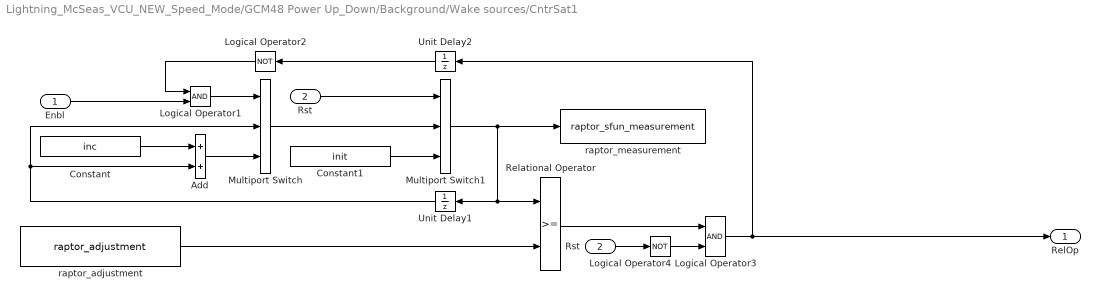
== system Lightning_McSeas_VCU_NEW_Speed_Mode/GCM48 Power Up_Down/Background/Wake sources/CntrSat1 ==
  Enbl : Inport
  Rst : Inport  Port=2
  Add : Sum  InputSameDT=on  OutDataTypeStr=Inherit: Same as first input
  Constant : Constant  Value=inc  OutDataTypeStr=uint32
  Constant1 : Constant  Value=init  OutDataTypeStr=uint32
  Logical Operator1 : Logic  OutDataTypeStr=boolean
  Logical Operator2 : Logic  Operator=NOT  Inputs=1  OutDataTypeStr=boolean
  Logical Operator3 : Logic  OutDataTypeStr=boolean
  Logical Operator4 : Logic  Operator=NOT  Inputs=1  OutDataTypeStr=boolean
  Multiport Switch : MultiPortSwitch  DataPortOrder=Zero-based contiguous  Inputs=2  zeroidx=on  InputSameDT=on
  Multiport Switch1 : MultiPortSwitch  DataPortOrder=Zero-based contiguous  Inputs=2  zeroidx=on  InputSameDT=on
  Relational Operator : RelationalOperator  OutDataTypeStr=boolean  RndMeth=Nearest
  "Rst " : InportShadow  Port=2
  Unit Delay1 : UnitDelay  InitialCondition=init  SampleTime=-1  HasFrameUpgradeWarning=on
  Unit Delay2 : UnitDelay  InitialCondition=boolean(0)  SampleTime=-1  HasFrameUpgradeWarning=on
  raptor_adjustment : Raptor_lib/Data Storage/raptor_adjustment  paramName=th_nam  nameSource=Parameter  initValue=5 / th_gain  dataType=uint32  storage=Calibration  calDispType=Number  calEnum={'Disabled', 'Enabled'}  calGain=th_gain  calOffset=0  calMax=inf  calMin=-inf  calFormat='0.3'  calUnit=th_units  calHelp=th_help  calAccess=4  calFunction=th_group  calDispHeaders=off  calColHeaders={'Col1' 'Col2' 'Col3'}  calRowHeaders={'Row1' 'Row2' 'Row3'}
      settings: SourceProductName=Raptor
  raptor_measurement : S-Function  FunctionName=raptor_sfun_measurement  Parameters=char({dataName,''}), uint8(calDispType), char(enumName), int32(enumValue), double(calGain), double(calOffset), double(calMax), double(calMin), char(calUnit), char(calHelp), char(calFormat), char(calFunction), char(calAccess)  SFunctionDeploymentMode=off  EnableBusSupport=off  mask(Measurement){paramName=[th_nam(1:end-3) 'Tmr'], nameSource=Parameter, calDispType=Number, calEnum={'False', 'True'}, calGain=th_gain, calOffset=0.0, calMax=inf, calMin=-inf, calFormat='0.3', calUnit=th_units, calHelp=['time that gets compared to ' th_nam], calAccess=4, calFunction=th_group, calVisible=on}
      mask prompts: paramName "Name"; nameSource "Name Source"; calDispType "Display as"; calEnum "Enumeration Definition"; calGain "Gain"; calOffset "Offset"; calMax "Max"; calMin "Min"; calFormat "Display Decimal Places"; calUnit "Unit Text"; calHelp "Help Text"; calAccess "Access Level"; calFunction "Function"; calVisible "Visible in Cal"
      mask help: This block is used to display a value in the calibration tool.
      mask init:
      | raptor_sfun_measurement_maskInit;
      settings: MoveFcn=raptor_icon_redraw(gcb);
      mask Help: eval('raptor_help(''raptor_measurement'');')
      mask TypeOptions nameSource: Parameter | Input Wire
      mask Callback nameSource: raptor_sfun_measurement_dlgCb(gcb, 'nameSource');
      mask TypeOptions calDispType: Number | Enumeration | String
      mask Callback calDispType: raptor_sfun_measurement_dlgCb(gcb, 'calDispType');
      mask TypeOptions calAccess: 4 | 3 | 2 | 1
      mask Display: raptor_sfun_measurement_icon;
  RelOp : Outport  VectorParamsAs1DForOutWhenUnconnected=off
  wires:
  "Rst "/1 -> Logical Operator4/1
  Logical Operator4/1 -> Logical Operator3/2
  Relational Operator/1 -> Logical Operator3/1
  Multiport Switch1/1 -> Relational Operator/1, Unit Delay1/1, raptor_measurement/1
  Logical Operator2/1 -> Logical Operator1/1
  Constant1/1 -> Multiport Switch1/3
  Multiport Switch/1 -> Multiport Switch1/2
  Constant/1 -> Add/1
  Unit Delay1/1 -> Multiport Switch/2, Add/2
  Add/1 -> Multiport Switch/3
  Logical Operator1/1 -> Multiport Switch/1
  Enbl/1 -> Logical Operator1/2
  raptor_adjustment/1 -> Relational Operator/2
  Logical Operator3/1 -> RelOp/1, Unit Delay2/1
  Rst/1 -> Multiport Switch1/1
  Unit Delay2/1 -> Logical Operator2/1

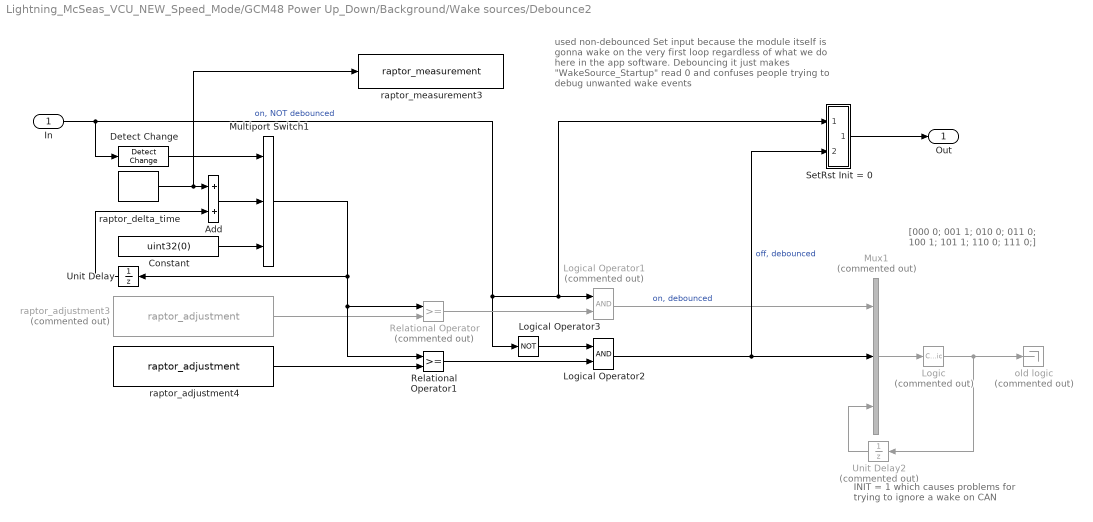
== system Lightning_McSeas_VCU_NEW_Speed_Mode/GCM48 Power Up_Down/Background/Wake sources/Debounce2 ==
  note: used non-debounced Set input because the module itself is gonna wake on the very first loop regardless of what we do here in the app software. Debouncing it just makes "WakeSource_Startup" read 0 and confuses people trying to debug unwanted wake events
  note: INIT = 1 which causes problems for trying to ignore a wake on CAN
  note: [000		0;
      |  001		1;
      |  010		0;
      |  011		0;
      |  100		1;
      |  101		1;
      |  110		0;
      |  111		0;]
  In : Inport
  Add : Sum
  Constant : Constant  Value=uint32(0)
  Detect Change : simulink/Logic and Bit Operations/Detect Change  vinit=0  OutDataTypeStr=boolean
  Logic : CombinatorialLogic  Commented=on  TruthTable=[0;1;0;0;1;1;0;0]
  Logical Operator1 : Logic  Commented=on  AllPortsSameDT=off  OutDataTypeStr=boolean
  Logical Operator2 : Logic  AllPortsSameDT=off  OutDataTypeStr=boolean
  Logical Operator3 : Logic  Operator=NOT  Inputs=1  AllPortsSameDT=off  OutDataTypeStr=boolean
  Multiport Switch1 : MultiPortSwitch  DataPortOrder=Zero-based contiguous  Inputs=2  zeroidx=on
  Mux1 : Mux  Commented=on  Inputs=3
  Relational Operator : RelationalOperator  Commented=on  OutDataTypeStr=boolean  RndMeth=Nearest
  Relational Operator1 : RelationalOperator  OutDataTypeStr=boolean  RndMeth=Nearest
  SetRst Init = 0 : Subsystem  mask(SetRst){init=0}
      mask prompts: init "Initial Condition (of output):"
      mask Display:
      | port_label('input', 1, 'S');
      | port_label('input', 2, 'R');
  Unit Delay : UnitDelay  InitialCondition=1  SampleTime=-1  HasFrameUpgradeWarning=on
  Unit Delay2 : UnitDelay  Commented=on  InitialCondition=1  SampleTime=-1  HasFrameUpgradeWarning=on
  old logic : Terminator  Commented=on
  raptor_adjustment3 : Raptor_lib/Data Storage/raptor_adjustment  Commented=on  paramName='KeySwHiTimeThr'  nameSource=Parameter  initValue=200  dataType=uint32  storage=Calibration  calDispType=Number  calEnum={'Active Low', 'Active High'}  calGain=1  calOffset=0  calMax=inf  calMin=-inf  calFormat='-1'  calUnit='milliseconds'  calHelp='State high time threshold'  calAccess=4  calFunction=group  calDispHeaders=off  calColHeaders={'Col1' 'Col2' 'Col3'}  calRowHeaders={'Row1' 'Row2' 'Row3'}
      settings: SourceProductName=Raptor
  raptor_adjustment4 : Raptor_lib/Data Storage/raptor_adjustment  paramName='KeySwLoTimeThr'  nameSource=Parameter  initValue=200  dataType=uint32  storage=Calibration  calDispType=Number  calEnum={'Active Low', 'Active High'}  calGain=1  calOffset=0  calMax=inf  calMin=-inf  calFormat='-1'  calUnit='milliseconds'  calHelp='State low time threshold'  calAccess=4  calFunction=group  calDispHeaders=off  calColHeaders={'Col1' 'Col2' 'Col3'}  calRowHeaders={'Row1' 'Row2' 'Row3'}
      settings: SourceProductName=Raptor
  raptor_delta_time : Raptor_lib/Triggers/raptor_delta_time  unit=milliseconds
      settings: SourceProductName=Raptor
  raptor_measurement3 : Raptor_lib/Data Storage/raptor_measurement  paramName='dt_read'  nameSource=Parameter  calDispType=Number  calEnum={'False', 'True'}  calGain=1.0  calOffset=0.0  calMax=inf  calMin=-inf  calFormat='-1'  calUnit=''  calHelp=''  calAccess=4  calFunction=group  calVisible=on
      settings: SourceProductName=Raptor
  Out : Outport  VectorParamsAs1DForOutWhenUnconnected=off
  wires:
  SetRst Init = 0/1(Bool) -> Out/1
  raptor_adjustment3/1 -> Relational Operator/2
  raptor_adjustment4/1 -> Relational Operator1/2
  raptor_delta_time/1 -> raptor_measurement3/1, Add/1
  Unit Delay/1 -> Add/2
  Logic/1 -> Unit Delay2/1, old logic/1
  Relational Operator1/1 -> Logical Operator2/2
  Constant/1 -> Multiport Switch1/3
  Add/1 -> Multiport Switch1/2
  Multiport Switch1/1 -> Relational Operator1/1, Relational Operator/1, Unit Delay/1
  In/1 -> Logical Operator3/1, Logical Operator1/1, SetRst Init = 0/1(Set), Detect Change/1  "on, NOT debounced"
  Unit Delay2/1 -> Mux1/3
  Mux1/1 -> Logic/1
  Logical Operator1/1 -> Mux1/1  "on, debounced"
  Logical Operator2/1 -> SetRst Init = 0/2(Rst), Mux1/2  "off, debounced"
  Relational Operator/1 -> Logical Operator1/2
  Logical Operator3/1 -> Logical Operator2/1
  Detect Change/1 -> Multiport Switch1/1

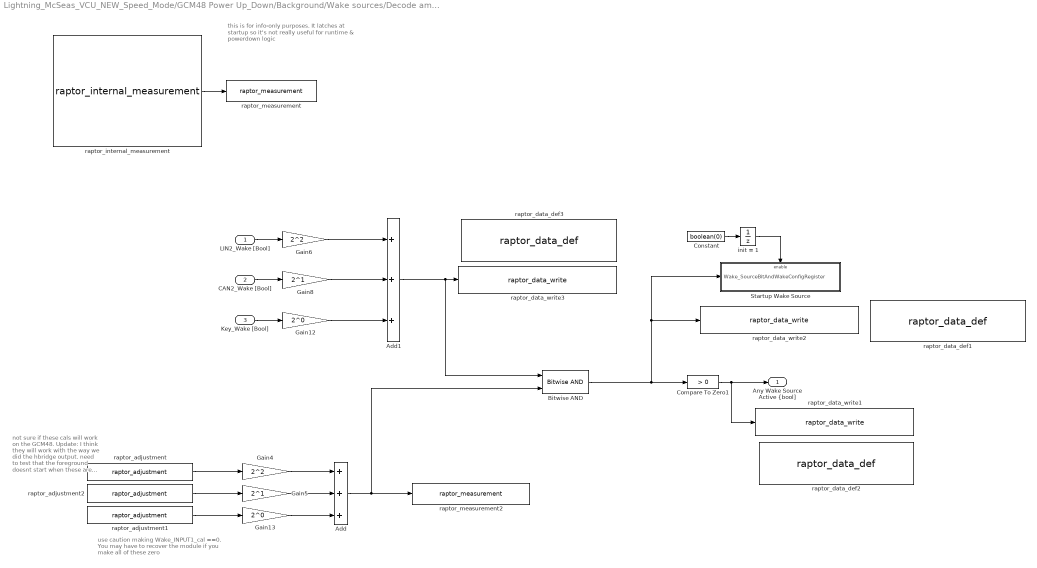
== system Lightning_McSeas_VCU_NEW_Speed_Mode/GCM48 Power Up_Down/Background/Wake sources/Decode amd Ignore Some Wake Sources ==
  note: this is for info-only purposes. It latches at startup so it's not really useful for runtime & powerdown logic
  note: not sure if these cals will work on the GCM48. Update: I think they will work with the way we did the hbridge output. need to test that the foreground doesnt start when these are zero
  note: use caution making Wake_INPUT1_cal ==0. You may have to recover the module if you make all of these zero
  LIN2_Wake [Bool] : Inport
  CAN2_Wake [Bool] : Inport  Port=2
  Key_Wake [Bool] : Inport  Port=3
  Add : Sum  Inputs=3  OutDataTypeStr=uint16
  Add1 : Sum  Inputs=3  OutDataTypeStr=uint16
  Bitwise AND : simulink/Logic and Bit Operations/Bitwise Operator  logicop=AND  UseBitMask=off  NumInputPorts=2  BitMask=bin2dec('11011001')  BitMaskRealWorld=Stored Integer
  Compare To Zero1 : simulink/Logic and Bit Operations/Compare To Zero  relop=>  OutDataTypeStr=boolean
  Constant : Constant  Value=boolean(0)
  Gain12 : Gain  Gain=2^0  OutDataTypeStr=uint16
  Gain13 : Gain  Gain=2^0  OutDataTypeStr=uint16
  Gain4 : Gain  Gain=2^2  OutDataTypeStr=uint16
  Gain5 : Gain  Gain=2^1  OutDataTypeStr=uint16
  Gain6 : Gain  Gain=2^2  OutDataTypeStr=uint16
  Gain8 : Gain  Gain=2^1  OutDataTypeStr=uint16
  Startup Wake Source : Subsystem  TreatAsAtomicUnit=on
  init = 1 : UnitDelay  InitialCondition=1  SampleTime=-1  HasFrameUpgradeWarning=on
  raptor_adjustment : Raptor_lib/Data Storage/raptor_adjustment  paramName='GCM48Wake_LIN2_cal'  nameSource=Parameter  initValue=0  dataType=boolean  storage=Calibration  calDispType=Number  calEnum={'False', 'True'}  calGain=1.0  calOffset=0.0  calMax=inf  calMin=-inf  calFormat='-1'  calUnit='bool'  calHelp='1 configures the module to wake via this input, 0 ignores this input'  calAccess=4  calFunction=group  calDispHeaders=off  calColHeaders={'Col1' 'Col2' 'Col3'}  calRowHeaders={'Row1' 'Row2' 'Row3'}
      settings: SourceProductName=Raptor
  raptor_adjustment1 : Raptor_lib/Data Storage/raptor_adjustment  paramName='GCM48Wake_INPUT1_cal'  nameSource=Parameter  initValue=1  dataType=boolean  storage=Calibration  calDispType=Number  calEnum={'False', 'True'}  calGain=1.0  calOffset=0.0  calMax=inf  calMin=-inf  calFormat='-1'  calUnit='bool'  calHelp='1 configures the module to wake via this input, 0 ignores this input'  calAccess=4  calFunction=group  calDispHeaders=off  calColHeaders={'Col1' 'Col2' 'Col3'}  calRowHeaders={'Row1' 'Row2' 'Row3'}
      settings: SourceProductName=Raptor
  raptor_adjustment2 : Raptor_lib/Data Storage/raptor_adjustment  paramName='GCM48Wake_CAN2_cal'  nameSource=Parameter  initValue=0  dataType=boolean  storage=Calibration  calDispType=Number  calEnum={'False', 'True'}  calGain=1.0  calOffset=0.0  calMax=inf  calMin=-inf  calFormat='-1'  calUnit='bool'  calHelp='1 configures the module to wake via this input, 0 ignores this input'  calAccess=4  calFunction=group  calDispHeaders=off  calColHeaders={'Col1' 'Col2' 'Col3'}  calRowHeaders={'Row1' 'Row2' 'Row3'}
      settings: SourceProductName=Raptor
  raptor_data_def1 : Raptor_lib/Data Storage/raptor_data_def  dataName='Wake_SourceBitAndWakeConfigRegister'  initValue=0  dataType=uint16  storage=Volatile (RAM)  calVisible=on  calType=Measurement  calDispType=Number  calEnum={'False', 'True'}  calGain=1.0  calOffset=0  calMin=-inf  calMax=inf  calFormat='-1'  calUnit=''  calHelp=''  calAccess=2  calFunction=group  calDispHeaders=off  calColHeaders={'Col1' 'Col2' 'Col3'}  calRowHeaders={'Row1' 'Row2' 'Row3'}
      settings: SourceProductName=Raptor
  raptor_data_def2 : Raptor_lib/Data Storage/raptor_data_def  dataName='Wake_AnyWakeSourceActive'  initValue=0  dataType=boolean  storage=Volatile (RAM)  calVisible=on  calType=Measurement  calDispType=Number  calEnum={'False', 'True'}  calGain=1.0  calOffset=0  calMin=-inf  calMax=inf  calFormat='-1'  calUnit='any wake source is keeping the module alive'  calHelp='bool'  calAccess=2  calFunction=group  calDispHeaders=off  calColHeaders={'Col1' 'Col2' 'Col3'}  calRowHeaders={'Row1' 'Row2' 'Row3'}
      settings: SourceProductName=Raptor
  raptor_data_def3 : Raptor_lib/Data Storage/raptor_data_def  dataName='WakeSource_Current'  initValue=0  dataType=uint16  storage=Volatile (RAM)  calVisible=on  calType=Measurement  calDispType=Number  calEnum={'False', 'True'}  calGain=1.0  calOffset=0  calMin=-inf  calMax=inf  calFormat='-1'  calUnit='wake source at the current instant'  calHelp=''  calAccess=2  calFunction=group  calDispHeaders=off  calColHeaders={'Col1' 'Col2' 'Col3'}  calRowHeaders={'Row1' 'Row2' 'Row3'}
      settings: SourceProductName=Raptor
  raptor_data_write1 : Raptor_lib/Data Storage/raptor_data_write  dataName='Wake_AnyWakeSourceActive'  dataShape=Scalar  idxSource=Input Port  idxRow=1  idxCol=1
      settings: SourceProductName=Raptor
  raptor_data_write2 : Raptor_lib/Data Storage/raptor_data_write  dataName='Wake_SourceBitAndWakeConfigRegister'  dataShape=Scalar  idxSource=Input Port  idxRow=1  idxCol=1
      settings: SourceProductName=Raptor
  raptor_data_write3 : Raptor_lib/Data Storage/raptor_data_write  dataName='WakeSource_Current'  dataShape=Scalar  idxSource=Input Port  idxRow=1  idxCol=1
      settings: SourceProductName=Raptor
  raptor_internal_measurement : Raptor_lib/Input & Output/raptor_internal_measurement  resourceValues=OUTPUT1_VFB|OUTPUT2_VFB|OUTPUT3_VFB|OUTPUT4_VFB|OUTPUT5_VFB|OUTPUT6_VFB|OUTPUT7_VFB|OUTPUT8_VFB|OUTPUT11_VFB|OUTPUT12_VFB|OUTPUT13_VFB|OUTPUT14_VFB|OUTPUT15_VFB|OUTPUT2_DFB|OUTPUT3_DFB|HBRIDGE9_10_DFB|OUTPUT2_IFB|OUTPUT3_IFB|HBRIDGE9_10_IFB|SENS_SUPPLY1_VFB|SENS_SUPPLY2_VFB|NTC_TEMP|WAKE_SOURCE|(None)  resource=WAKE_SOURCE  out_eng=0  soft_filter=1  out_bool=0
      settings: SourceProductName=Raptor
  raptor_measurement : Raptor_lib/Data Storage/raptor_measurement  paramName='WakeSource_RaptorIntrnlMeas'  nameSource=Parameter  calDispType=Number  calEnum={'False', 'True'}  calGain=1.0  calOffset=0.0  calMax=inf  calMin=-inf  calFormat='-1'  calUnit='wake source at startup... kinda. it often reads that LIN work the module even if the LIN bus isnt connected.'  calHelp=''  calAccess=4  calFunction=group  calVisible=on
      settings: SourceProductName=Raptor
  raptor_measurement2 : Raptor_lib/Data Storage/raptor_measurement  paramName='WakeConfigRegister'  nameSource=Parameter  calDispType=Number  calEnum={'False', 'True'}  calGain=1.0  calOffset=0.0  calMax=inf  calMin=-inf  calFormat='-1'  calUnit='register'  calHelp=''  calAccess=4  calFunction=group  calVisible=on
      settings: SourceProductName=Raptor
  "Any Wake Source Active {bool]" : Outport  VectorParamsAs1DForOutWhenUnconnected=off
  wires:
  Key_Wake [Bool]/1 -> Gain12/1
  init = 1/1 -> Startup Wake Source/Enable
  Constant/1 -> init = 1/1
  Compare To Zero1/1 -> "Any Wake Source Active {bool]"/1, raptor_data_write1/1
  LIN2_Wake [Bool]/1 -> Gain6/1
  CAN2_Wake [Bool]/1 -> Gain8/1
  raptor_adjustment1/1 -> Gain13/1
  Gain13/1 -> Add/3
  Gain12/1 -> Add1/3
  Add1/1 -> raptor_data_write3/1, Bitwise AND/1
  Gain6/1 -> Add1/1
  Gain8/1 -> Add1/2
  Bitwise AND/1 -> raptor_data_write2/1, Startup Wake Source/1(Wake_SourceBitAndWakeConfigRegister), Compare To Zero1/1
  raptor_adjustment2/1 -> Gain5/1
  Gain5/1 -> Add/2
  Add/1 -> raptor_measurement2/1, Bitwise AND/2
  raptor_internal_measurement/1 -> raptor_measurement/1
  raptor_adjustment/1 -> Gain4/1
  Gain4/1 -> Add/1

== system Lightning_McSeas_VCU_NEW_Speed_Mode/GCM48 Power Up_Down/Background/Wake sources/Dtc ==
  In : Inport
  Delay Input1 : UnitDelay  Description=Store in Global RAM  DisableCoverage=on  InitialCondition=init  SampleTime=-1  HasFrameUpgradeWarning=on
  Relational Operator : RelationalOperator  Operator===  OutDataTypeStr=boolean  RndMeth=Nearest  InputSameDT=on
  Bool : Outport  InitialOutput=0  VectorParamsAs1DForOutWhenUnconnected=off
  wires:
  In/1 -> Delay Input1/1, Relational Operator/1
  Delay Input1/1 -> Relational Operator/2
  Relational Operator/1 -> Bool/1

== system Lightning_McSeas_VCU_NEW_Speed_Mode/GCM48 Power Up_Down/Background/Wake sources/Dtc1 ==
  In : Inport
  Delay Input1 : UnitDelay  Description=Store in Global RAM  DisableCoverage=on  InitialCondition=init  SampleTime=-1  HasFrameUpgradeWarning=on
  Relational Operator : RelationalOperator  Operator===  OutDataTypeStr=boolean  RndMeth=Nearest  InputSameDT=on
  Bool : Outport  InitialOutput=0  VectorParamsAs1DForOutWhenUnconnected=off
  wires:
  Relational Operator/1 -> Bool/1
  Delay Input1/1 -> Relational Operator/2
  In/1 -> Relational Operator/1, Delay Input1/1

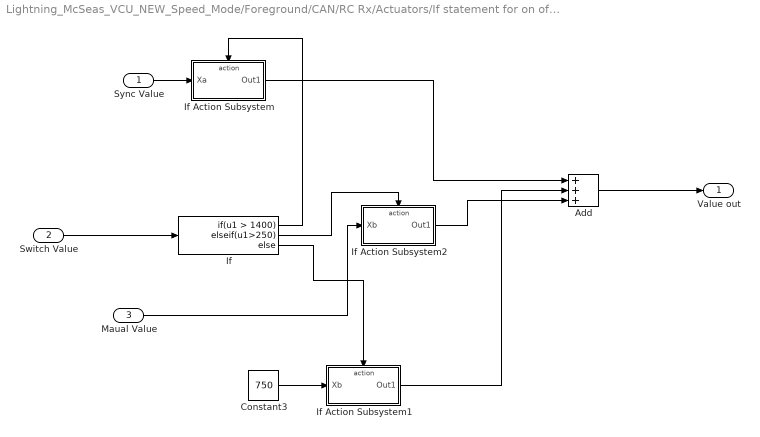
== system Lightning_McSeas_VCU_NEW_Speed_Mode/Foreground/CAN/RC Rx/Actuators/If statement for on off switch1 ==
  Sync Value : Inport
  Switch Value : Inport  Port=2
  Maual Value : Inport  Port=3
  Add : Sum  Inputs=+++
  Constant3 : Constant  Value=750
  If : If  IfExpression=u1 > 1400  ElseIfExpressions=u1>250
  If Action Subsystem : Subsystem  TreatAsAtomicUnit=on
  If Action Subsystem1 : Subsystem  TreatAsAtomicUnit=on
  If Action Subsystem2 : Subsystem  TreatAsAtomicUnit=on
  Value out : Outport
  wires:
  If/3 -> If Action Subsystem1/Action
  Switch Value/1 -> If/1
  Sync Value/1 -> If Action Subsystem/1(Xa)
  If Action Subsystem1/1(Out1) -> Add/2
  Add/1 -> Value out/1
  If/1 -> If Action Subsystem/Action
  Constant3/1 -> If Action Subsystem1/1(Xb)
  If Action Subsystem/1(Out1) -> Add/1
  If/2 -> If Action Subsystem2/Action
  If Action Subsystem2/1(Out1) -> Add/3
  Maual Value/1 -> If Action Subsystem2/1(Xb)

== system Lightning_McSeas_VCU_NEW_Speed_Mode/Foreground/CAN/RC Rx/Actuators/Subsystem ==
  Front left : Inport
  Rise of Front : Inport  Port=2
  Gain : Gain  Gain=1/1500
  Product : Product
  Actuator value : Outport
  wires:
  Front left/1 -> Gain/1
  Rise of Front/1 -> Product/1
  Gain/1 -> Product/2
  Product/1 -> Actuator value/1

== system Lightning_McSeas_VCU_NEW_Speed_Mode/Foreground/CAN/RC Rx/Battery Charging/Inverter ==
  note: 0 = Charging
      | 1 = STOP
  In1 : Inport
  Constant : Constant  Value=0
  Constant1 : Constant
  If : If
  If Action Subsystem : Subsystem  TreatAsAtomicUnit=on
  If Action Subsystem1 : Subsystem  TreatAsAtomicUnit=on
  Merge : Merge
  Out1 : Outport
  wires:
  In1/1 -> If/1
  If/1 -> If Action Subsystem/Action
  If/2 -> If Action Subsystem1/Action
  Constant/1 -> If Action Subsystem/1(In1)
  Constant1/1 -> If Action Subsystem1/1(In1)
  If Action Subsystem/1(Out1) -> Merge/1
  If Action Subsystem1/1(Out1) -> Merge/2
  Merge/1 -> Out1/1
